simulink model "Simulink_Deliverable1_2__2_"  (R2025b)
settings: Solver=FixedStepAuto  StartTime=0.0  StopTime=10.0  FixedStep=1e-3  RelTol=1e-3  EnableMultiTasking=on
undefined symbols (not defined in the file): A0, A1, A2, A3, A4, D0, D1, D10, D11, D12, D13, D2, D3, D4, D5, D6, D7, D8, D9, PTA0, PTA1, PTA2, PTB10, PTB11, PTB2, PTB23, PTB3, PTB9, PTC11, PTC16, PTC17, PTC2, PTC3, PTC4, PTD0, PTD1, PTD2, PTD3
libraries: frdmk64flib x22, etargetslib x6, dspstat3 x2
settings Model: ExtModeTrigDuration=5  Creator=shaun  LastModifiedBy=anila
settings OptimizationCC: DefaultParameterBehavior=Inlined  EnhancedBackFolding=on  PassReuseOutputArgsAs=Individual arguments  ZeroExternalMemoryAtStartup=off  ZeroInternalMemoryAtStartup=off  MaxStackSize=64  OptimizeBlockOrder=speed  DifferentSizesBufferReuse=on  OptimizationCustomize=off  EfficientTunableParamExpr=on
settings DebuggingCC: ParameterTunabilityLossMsg=error
settings HardwareCC: ProdBitPerPointer=32.0  ProdBitPerSizeT=32.0  ProdBitPerPtrDiffT=32.0  ProdLargestAtomicInteger=Long  ProdLargestAtomicFloat=Double  ProdWordSize=32.0  ProdHWDeviceType=ARM Compatible->ARM Cortex
settings SFSimCC: MATLABDynamicMemAlloc=off
settings RTWCC: SystemTargetFile=ert.tlc  HardwareBoard=NXP FRDM-K64F  TLCOptions="-aInlineSetEventsForThisBaseRateFcn=TLC_FALSE -aSuppressMultiTaskScheduler=TLC_FALSE  -aRateBasedStepFcn=0"  TemplateMakefile=ert_default_tmf  Toolchain=GNU Tools for ARM Embedded Processors  Description=Embedded Coder
settings CodeAppCC: ForceParamTrailComments=on  IgnoreCustomStorageClasses=off  OperatorAnnotations=on  SimulinkDataObjDesc=on  SFDataObjDesc=on  InsertBlockDesc=on
settings ERTTargetCC: ExtModeTransport=4.0  ExtModeMexFile=sendToCommService

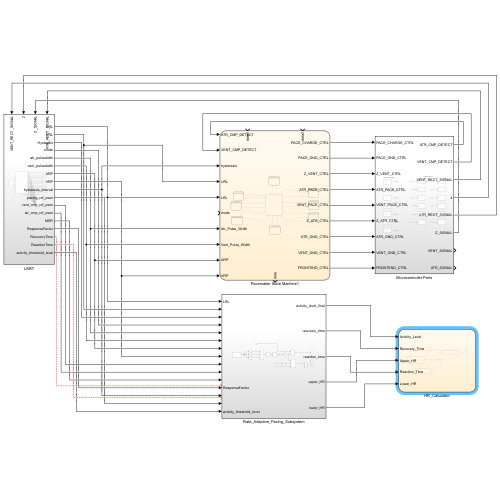
[thumbnail: Simulink's stored preview of the top-level diagram]
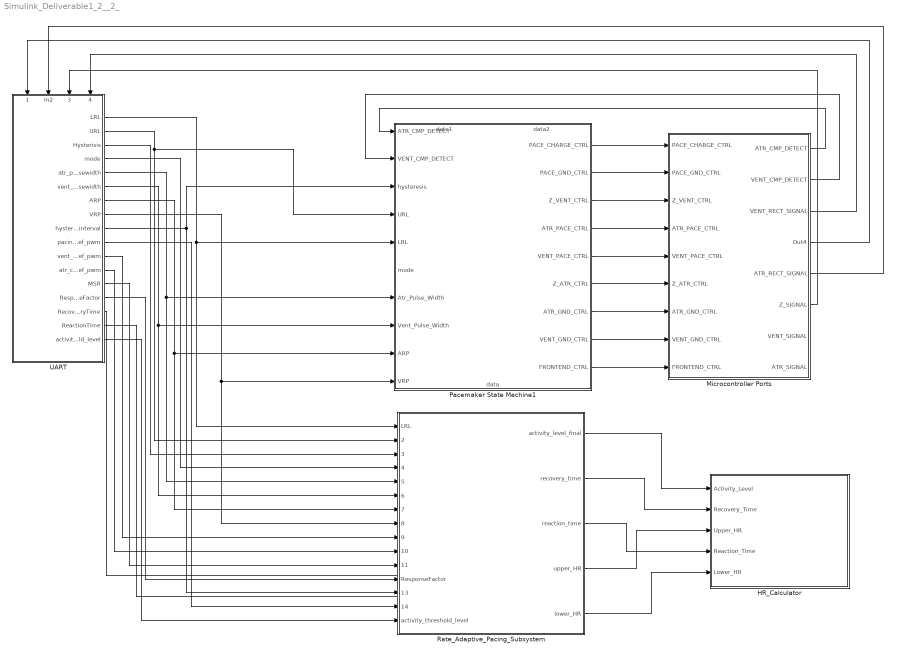
== system Simulink_Deliverable1_2__2_ ==
  HR_Calculator : Stateflow chart  TreatAsAtomicUnit=on
      settings: PortSchema="{\"entries\":[{\"content\":{\"sides\":[{\"content\":{\"connectorIds\":[\"In5\",\"In2\",\"In3\",\"In4\",\"In1\"]},\"type\":\"ConnectorPlacement.EquallySpacedRectSide\",\"uuid\":\"4fd71a97-0d96-44cf-9a3b-b475d577ae04\"},{\"content\":{\"side\":\"RIGHT\"},\"type\":\"ConnectorPlacement.EquallySpacedRectSide\",\"uuid\":\"faba256d-fac9-4ab5-bd75-12f2978d4ab7\"},{\"content\":{\"side\":\"TOP\"},\"type\":\"ConnectorPlacement.EquallySpacedRectSide\",\"uuid\":\"a02d704a-be11-4cb0-b416-0f22440acd8a\"}]},\"type\":\"ConnectorPlacement.EquallySpacedConnector\",\"uuid\":\"fcc24184-24f4-4090-bbbe-791745e2298d\"}],\"packageUris\":[\"http://schema.mathworks.com/mf0/Connector/R2020b\"],\"version\":\"1.0\"}"
  Microcontroller Ports : Subsystem
  Pacemaker State Machine1 : Stateflow chart  TreatAsAtomicUnit=on
      settings: PortSchema="{\"entries\":[{\"content\":{\"sides\":[{\"content\":{\"connectorIds\":[\"In4\",\"In11\",\"In3\",\"In5\",\"In6\",\"In9\",\"In7\",\"In10\",\"In8\",\"In12\"]},\"type\":\"ConnectorPlacement.EquallySpacedRectSide\",\"uuid\":\"3d18841d-ac72-4031-8466-622516bc8e89\"},{\"content\":{\"connectorIds\":[\"Out5\",\"Out6\",\"Out10\",\"Out3\",\"Out8\",\"Out9\",\"Out2\",\"Out7\",\"Out4\"],\"side\":\"RIGHT\"},\"type\":\"ConnectorPlacement.EquallySpacedRectSide\",\"uuid\":\"4d13c4f7-6767-44e3-9325-4ac8cd89e11a\"},{\"content\":{\"connectorIds\":[\"In1\",\"In2\"],\"side\":\"TOP\"},\"type\":\"ConnectorPlacement.EquallySpacedRectSide\",\"uuid\":\"87410120-6407-4e47-b91e-6c9b7b921b96\"},{\"content\":{\"connectorIds\":[\"Out1\"],\"side\":\"BOTTOM\"},\"type\":\"ConnectorPlacement.EquallySpacedRectSide\",\"uuid\":\"b376cdcd-045a-4cf2-9c04-75ec87224bb6\"}]},\"type\":\"ConnectorPlacement.EquallySpacedConnector\",\"uuid\":\"fed7b079-bf69-4c2d-9ed3-910cc0ad36be\"}],\"packageUris\":[\"http://schema.mathworks.com/mf0/Connector/R2020b\"],\"version\":\"1.0\"}"
  Rate_Adaptive_Pacing_Subsystem : Subsystem
  UART : Subsystem
      settings: PortSchema="{\"entries\":[{\"content\":{\"sides\":[{\"content\":{},\"type\":\"ConnectorPlacement.EquallySpacedRectSide\",\"uuid\":\"183065aa-c741-4563-b5ae-3020154dfd83\"},{\"content\":{\"connectorIds\":[\"Out1\",\"Out2\",\"Out3\",\"Out4\",\"Out5\",\"Out6\",\"Out7\",\"Out8\",\"Out9\",\"Out10\",\"Out11\",\"Out12\",\"Out13\",\"Out14\",\"Out15\",\"Out16\",\"Out17\"],\"side\":\"RIGHT\"},\"type\":\"ConnectorPlacement.EquallySpacedRectSide\",\"uuid\":\"65727c57-e161-4cba-a0e8-016175ec1656\"},{\"content\":{\"connectorIds\":[\"In1\",\"In2\",\"In3\",\"In4\"],\"side\":\"TOP\"},\"type\":\"ConnectorPlacement.EquallySpacedRectSide\",\"uuid\":\"c897ad8a-6ebd-4b90-9657-b8410c3521bd\"}]},\"type\":\"ConnectorPlacement.EquallySpacedConnector\",\"uuid\":\"08bd3836-6b13-4613-84df-35379265e920\"}],\"packageUris\":[\"http://schema.mathworks.com/mf0/Connector/R2020b\"],\"version\":\"1.0\"}"
  wires:
  Microcontroller Ports/2(VENT_CMP_DETECT) -> Pacemaker State Machine1/11(VENT_CMP_DETECT)
  Pacemaker State Machine1/9(Z_ATR_CTRL) -> Microcontroller Ports/6(Z_ATR_CTRL)
  Pacemaker State Machine1/4(FRONTEND_CTRL) -> Microcontroller Ports/9(FRONTEND_CTRL)
  Pacemaker State Machine1/5(PACE_CHARGE_CTRL) -> Microcontroller Ports/1(PACE_CHARGE_CTRL)
  Pacemaker State Machine1/3(ATR_PACE_CTRL) -> Microcontroller Ports/4(ATR_PACE_CTRL)
  Pacemaker State Machine1/2(ATR_GND_CTRL) -> Microcontroller Ports/7(ATR_GND_CTRL)
  Microcontroller Ports/1(ATR_CMP_DETECT) -> Pacemaker State Machine1/4(ATR_CMP_DETECT)
  Pacemaker State Machine1/8(VENT_PACE_CTRL) -> Microcontroller Ports/5(VENT_PACE_CTRL)
  Pacemaker State Machine1/6(PACE_GND_CTRL) -> Microcontroller Ports/2(PACE_GND_CTRL)
  Pacemaker State Machine1/10(Z_VENT_CTRL) -> Microcontroller Ports/3(Z_VENT_CTRL)
  Pacemaker State Machine1/7(VENT_GND_CTRL) -> Microcontroller Ports/8(VENT_GND_CTRL)
  UART/7(ARP) -> Pacemaker State Machine1/8(ARP), Rate_Adaptive_Pacing_Subsystem/7
  UART/5(atr_pulsewidth) -> Pacemaker State Machine1/7(Atr_Pulse_Width), Rate_Adaptive_Pacing_Subsystem/5
  UART/17(activity_threshold_level) -> Rate_Adaptive_Pacing_Subsystem/15(activity_threshold_level)
  UART/14(ResponseFactor) -> Rate_Adaptive_Pacing_Subsystem/12(ResponseFactor)
  UART/1(LRL) -> Pacemaker State Machine1/6(LRL), Rate_Adaptive_Pacing_Subsystem/1(LRL)
  UART/15(RecoveryTime) -> ?
  UART/16(ReactionTime) -> ?
  UART/2(URL) -> Pacemaker State Machine1/5(URL), Rate_Adaptive_Pacing_Subsystem/2
  UART/3(Hysterisis) -> Rate_Adaptive_Pacing_Subsystem/3
  UART/4(mode) -> Rate_Adaptive_Pacing_Subsystem/4
  UART/6(vent_pulsewidth) -> Pacemaker State Machine1/10(Vent_Pulse_Width), Rate_Adaptive_Pacing_Subsystem/6
  UART/8(VRP) -> Pacemaker State Machine1/12(VRP), Rate_Adaptive_Pacing_Subsystem/8
  UART/9(hysteresis_interval) -> Pacemaker State Machine1/3(hysteresis), Rate_Adaptive_Pacing_Subsystem/13
  UART/10(pacing_ref_pwm) -> Rate_Adaptive_Pacing_Subsystem/14
  UART/11(vent_cmp_ref_pwm) -> Rate_Adaptive_Pacing_Subsystem/9
  UART/12(atr_cmp_ref_pwm) -> Rate_Adaptive_Pacing_Subsystem/10
  UART/13(MSR) -> Rate_Adaptive_Pacing_Subsystem/11
  Rate_Adaptive_Pacing_Subsystem/5(lower_HR) -> HR_Calculator/1(Lower_HR)
  Rate_Adaptive_Pacing_Subsystem/1(activity_level_final) -> HR_Calculator/5(Activity_Level)
  Rate_Adaptive_Pacing_Subsystem/2(recovery_time) -> HR_Calculator/2(Recovery_Time)
  Rate_Adaptive_Pacing_Subsystem/4(upper_HR) -> HR_Calculator/3(Upper_HR)
  Rate_Adaptive_Pacing_Subsystem/3(reaction_time) -> HR_Calculator/4(Reaction_Time)
  Microcontroller Ports/3(VENT_RECT_SIGNAL) -> UART/4(ATR_RECT_SIGNAL)
  Microcontroller Ports/4(Out4) -> UART/1(VENT_RECT_SIGNAL)
  Microcontroller Ports/5(ATR_RECT_SIGNAL) -> UART/2(In2)
  Microcontroller Ports/6(Z_SIGNAL) -> UART/3(Z_SIGNAL)

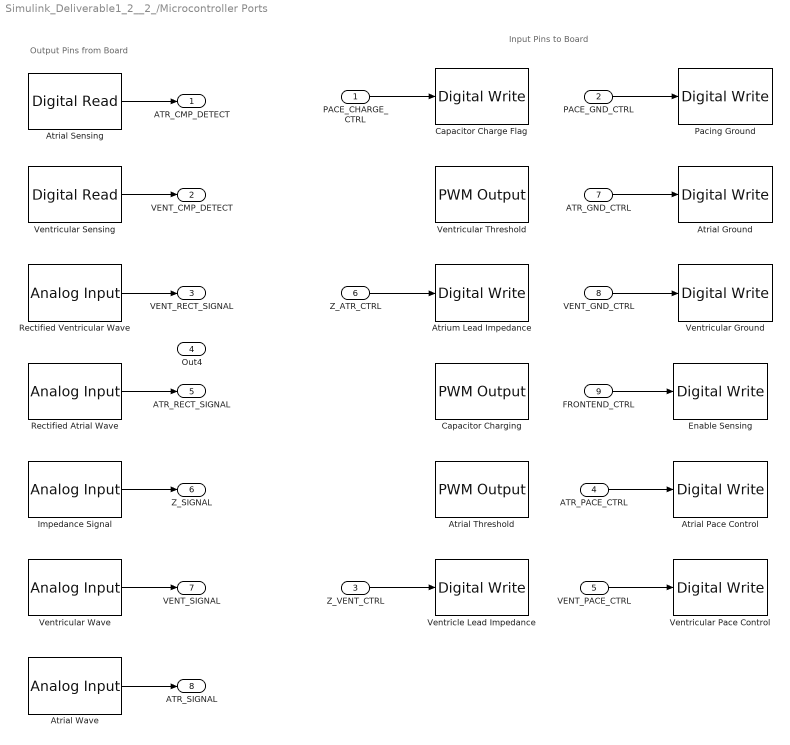
== system Simulink_Deliverable1_2__2_/Microcontroller Ports ==
  note: Output Pins from Board
  note: Input Pins to Board
  PACE_CHARGE_CTRL : Inport
  PACE_GND_CTRL : Inport  Port=2
  Z_VENT_CTRL : Inport  Port=3
  ATR_PACE_CTRL : Inport  Port=4
  VENT_PACE_CTRL : Inport  Port=5
  Z_ATR_CTRL : Inport  Port=6
  ATR_GND_CTRL : Inport  Port=7
  VENT_GND_CTRL : Inport  Port=8
  FRONTEND_CTRL : Inport  Port=9
  Atrial Ground : frdmk64flib/Digital Write  Whichpin=PTD2 (D11)
  Atrial Pace Control : frdmk64flib/Digital Write  Whichpin=PTA0 (D8)
  Atrial Sensing : frdmk64flib/Digital Read  Whichpin=PTC16 (D0)  SampleTime=-1
  Atrial Threshold : frdmk64flib/PWM Output  Whichpin=PTC2 (D6)  InitialFrequency=2000  InitialDutyCycle=0
  Atrial Wave : frdmk64flib/Analog Input  Whichpin=PTB2 (A0)  SampleTime=-1
  Atrium Lead Impedance : frdmk64flib/Digital Write  Whichpin=PTB23 (D4)
  Capacitor Charge Flag : frdmk64flib/Digital Write  Whichpin=PTB9 (D2)
  Capacitor Charging : frdmk64flib/PWM Output  Whichpin=PTA2 (D5)  InitialFrequency=2000  InitialDutyCycle=0
  Enable Sensing : frdmk64flib/Digital Write  Whichpin=PTD1 (D13)
  Impedance Signal : frdmk64flib/Analog Input  Whichpin=PTB10 (A2)  SampleTime=-1
  Pacing Ground : frdmk64flib/Digital Write  Whichpin=PTD0 (D10)
  Rectified Atrial Wave : frdmk64flib/Analog Input  Whichpin=PTB11 (A3)  SampleTime=-1
  Rectified Ventricular Wave : frdmk64flib/Analog Input  Whichpin=PTC11 (A4)  SampleTime=-1
  Ventricle Lead Impedance : frdmk64flib/Digital Write  Whichpin=PTC3 (D7)
  Ventricular Ground : frdmk64flib/Digital Write  Whichpin=PTD3 (D12)
  Ventricular Pace Control : frdmk64flib/Digital Write  Whichpin=PTC4 (D9)
  Ventricular Sensing : frdmk64flib/Digital Read  Whichpin=PTC17 (D1)  SampleTime=-1
  Ventricular Threshold : frdmk64flib/PWM Output  Whichpin=PTA1 (D3)  InitialFrequency=2000  InitialDutyCycle=0
  Ventricular Wave : frdmk64flib/Analog Input  Whichpin=PTB3 (A1)  SampleTime=-1
  ATR_CMP_DETECT : Outport
  VENT_CMP_DETECT : Outport  Port=2
  VENT_RECT_SIGNAL : Outport  Port=3
  Out4 : Outport  Port=4
  ATR_RECT_SIGNAL : Outport  Port=5
  Z_SIGNAL : Outport  Port=6
  VENT_SIGNAL : Outport  Port=7
  ATR_SIGNAL : Outport  Port=8
  wires:
  Atrial Sensing/1 -> ATR_CMP_DETECT/1
  Ventricular Sensing/1 -> VENT_CMP_DETECT/1
  PACE_CHARGE_CTRL/1 -> Capacitor Charge Flag/1
  ? -> Ventricular Threshold/1
  Z_ATR_CTRL/1 -> Atrium Lead Impedance/1
  ? -> Capacitor Charging/1
  ? -> Atrial Threshold/1
  Z_VENT_CTRL/1 -> Ventricle Lead Impedance/1
  ATR_PACE_CTRL/1 -> Atrial Pace Control/1
  VENT_PACE_CTRL/1 -> Ventricular Pace Control/1
  PACE_GND_CTRL/1 -> Pacing Ground/1
  ATR_GND_CTRL/1 -> Atrial Ground/1
  VENT_GND_CTRL/1 -> Ventricular Ground/1
  FRONTEND_CTRL/1 -> Enable Sensing/1
  Rectified Atrial Wave/1 -> ATR_RECT_SIGNAL/1
  Rectified Ventricular Wave/1 -> VENT_RECT_SIGNAL/1
  Impedance Signal/1 -> Z_SIGNAL/1
  Ventricular Wave/1 -> VENT_SIGNAL/1
  Atrial Wave/1 -> ATR_SIGNAL/1

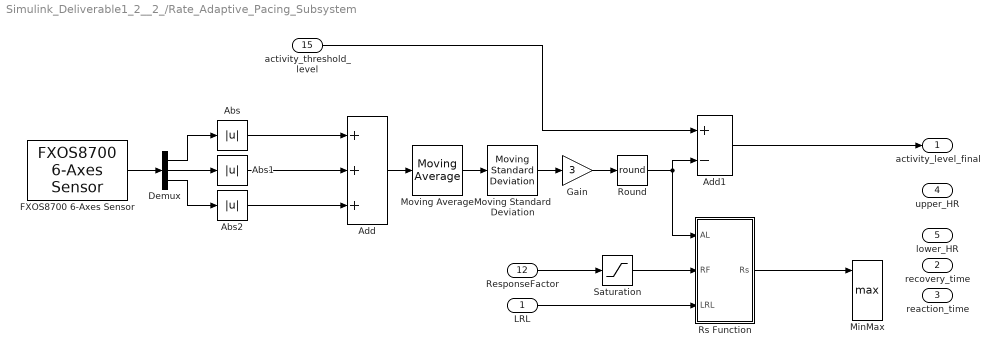
== system Simulink_Deliverable1_2__2_/Rate_Adaptive_Pacing_Subsystem ==
  LRL : Inport
  ResponseFactor : Inport  Port=12
  activity_threshold_level : Inport  Port=15
  Abs : Abs  SaturateOnIntegerOverflow=off
  Abs1 : Abs  SaturateOnIntegerOverflow=off
  Abs2 : Abs  SaturateOnIntegerOverflow=off
  Add : Sum  Inputs=+++
  Add1 : Sum  Inputs=+-
  Demux : Demux  Outputs=3
  FXOS8700 6-Axes Sensor : frdmk64flib/FXOS8700 6-Axes Sensor  Activesensor=Accelerometer only  ODR=800Hz  HybridODR=400Hz  Accelfullrange=-4g to +4g  SampleTime=-1
  Gain : Gain  Gain=3
  MinMax : MinMax  Function=max  Inputs=3
  Moving Average : dspstat3/Moving Average  Method=Sliding window  ForgettingFactorPort=off  SpecifyWindowLength=on  WindowLength=4  OverlapLength=3  AllowArbitraryInputLength=off  ForgettingFactor=0.9  SimulateUsing=Interpreted execution
  Moving Standard Deviation : dspstat3/Moving Standard Deviation  Method=Sliding window  ForgettingFactorPort=off  SpecifyWindowLength=on  WindowLength=4  OverlapLength=3  AllowArbitraryInputLength=off  ForgettingFactor=0.9  SimulateUsing=Interpreted execution
  Round : Rounding  Operator=round
  Rs Function : MATLAB Function  TreatAsAtomicUnit=on
  Saturation : Saturate  UpperLimit=14
  activity_level_final : Outport
  recovery_time : Outport  Port=2
  reaction_time : Outport  Port=3
  upper_HR : Outport  Port=4
  lower_HR : Outport  Port=5
  wires:
  FXOS8700 6-Axes Sensor/1 -> Demux/1
  Demux/1 -> Abs/1
  Demux/2 -> Abs1/1
  Demux/3 -> Abs2/1
  Abs/1 -> Add/1
  Abs1/1 -> Add/2
  Abs2/1 -> Add/3
  Add/1 -> Moving Average/1
  Moving Average/1 -> Moving Standard Deviation/1
  Moving Standard Deviation/1 -> Gain/1
  Gain/1 -> Round/1
  Round/1 -> Rs Function/1(AL), Add1/2
  LRL/1 -> Rs Function/3(LRL)
  Saturation/1 -> Rs Function/2(RF)
  ResponseFactor/1 -> Saturation/1
  activity_threshold_level/1 -> Add1/1
  Add1/1 -> activity_level_final/1
  Rs Function/1(Rs) -> MinMax/1

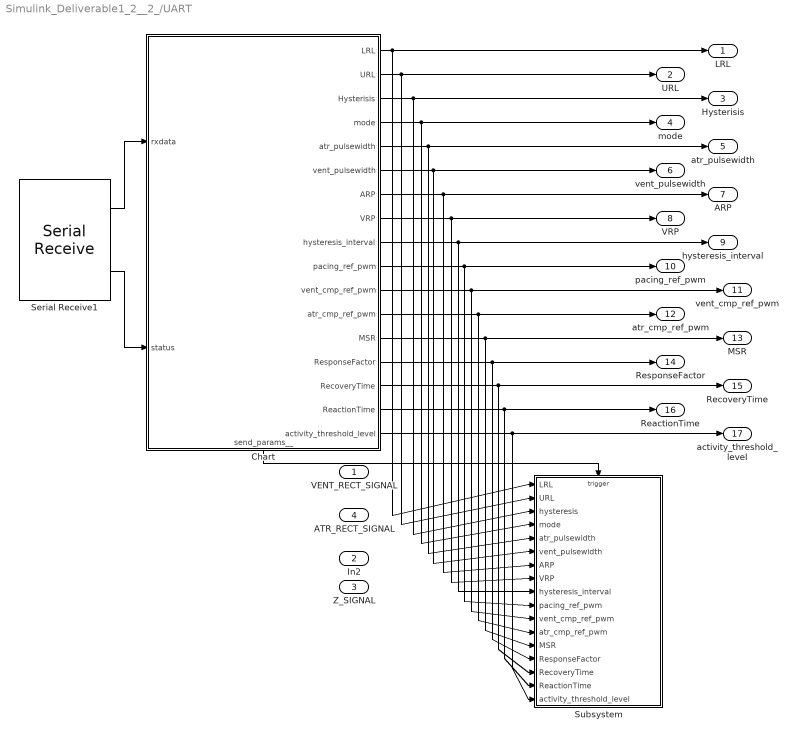
== system Simulink_Deliverable1_2__2_/UART ==
  VENT_RECT_SIGNAL : Inport
  In2 : Inport  Port=2
  Z_SIGNAL : Inport  Port=3
  ATR_RECT_SIGNAL : Inport  Port=4
  Chart : Stateflow chart  TreatAsAtomicUnit=on
      settings: PortSchema="{\"entries\":[{\"content\":{\"sides\":[{\"content\":{\"connectorIds\":[\"In1\",\"In2\"]},\"type\":\"ConnectorPlacement.EquallySpacedRectSide\",\"uuid\":\"bebe3e22-0960-44d0-8399-67e14216072d\"},{\"content\":{\"connectorIds\":[\"Out2\",\"Out3\",\"Out4\",\"Out5\",\"Out6\",\"Out7\",\"Out8\",\"Out9\",\"Out10\",\"Out11\",\"Out12\",\"Out13\",\"Out14\",\"Out15\",\"Out16\",\"Out17\",\"Out18\"],\"side\":\"RIGHT\"},\"type\":\"ConnectorPlacement.EquallySpacedRectSide\",\"uuid\":\"a4088612-4ea4-4c29-88bf-96f9d2b4fd9c\"},{\"content\":{\"side\":\"TOP\"},\"type\":\"ConnectorPlacement.EquallySpacedRectSide\",\"uuid\":\"7904bd59-2d39-416f-99c6-ab75130198a6\"},{\"content\":{\"connectorIds\":[\"Out1\"],\"side\":\"BOTTOM\"},\"type\":\"ConnectorPlacement.EquallySpacedRectSide\",\"uuid\":\"eb209d23-bc9c-4e28-840d-c030bd2810ba\"}]},\"type\":\"ConnectorPlacement.EquallySpacedConnector\",\"uuid\":\"1093a67f-4a83-45ff-8a38-c0bee63203db\"}],\"packageUris\":[\"http://schema.mathworks.com/mf0/Connector/R2020b\"],\"version\":\"1.0\"}"
  Serial Receive1 : frdmk64flib/Serial Receive  SCIModule=0  Baudrate=uint32(9600)  Parity=None  StopBits=1  HardwareFlowControl=None  ByteOrder=LittleEndian  DataType=uint8  DataLength=10  BlockingMode=off  OutputStatus=on  SampleTime=-1
  Subsystem : Subsystem
  LRL : Outport
  URL : Outport  Port=2
  Hysterisis : Outport  Port=3
  mode : Outport  Port=4
  atr_pulsewidth : Outport  Port=5
  vent_pulsewidth : Outport  Port=6
  ARP : Outport  Port=7
  VRP : Outport  Port=8
  hysteresis_interval : Outport  Port=9
  pacing_ref_pwm : Outport  Port=10
  vent_cmp_ref_pwm : Outport  Port=11
  atr_cmp_ref_pwm : Outport  Port=12
  MSR : Outport  Port=13
  ResponseFactor : Outport  Port=14
  RecoveryTime : Outport  Port=15
  ReactionTime : Outport  Port=16
  activity_threshold_level : Outport  Port=17
  wires:
  Serial Receive1/1 -> Chart/1(rxdata)
  Serial Receive1/2 -> Chart/2(status)
  Chart/2(LRL) -> LRL/1, Subsystem/1(LRL)
  Chart/3(URL) -> URL/1, Subsystem/2(URL)
  Chart/4(Hysterisis) -> Subsystem/3(hysteresis), Hysterisis/1
  Chart/5(mode) -> Subsystem/4(mode), mode/1
  Chart/6(atr_pulsewidth) -> Subsystem/5(atr_pulsewidth), atr_pulsewidth/1
  Chart/7(vent_pulsewidth) -> Subsystem/6(vent_pulsewidth), vent_pulsewidth/1
  Chart/8(ARP) -> Subsystem/7(ARP), ARP/1
  Chart/9(VRP) -> Subsystem/8(VRP), VRP/1
  Chart/10(hysteresis_interval) -> Subsystem/9(hysteresis_interval), hysteresis_interval/1
  Chart/11(pacing_ref_pwm) -> Subsystem/10(pacing_ref_pwm), pacing_ref_pwm/1
  Chart/12(vent_cmp_ref_pwm) -> Subsystem/11(vent_cmp_ref_pwm), vent_cmp_ref_pwm/1
  Chart/13(atr_cmp_ref_pwm) -> Subsystem/12(atr_cmp_ref_pwm), atr_cmp_ref_pwm/1
  Chart/14(MSR) -> Subsystem/13(MSR), MSR/1
  Chart/15(ResponseFactor) -> Subsystem/14(ResponseFactor), ResponseFactor/1
  Chart/16(RecoveryTime) -> Subsystem/15(RecoveryTime), RecoveryTime/1
  Chart/17(ReactionTime) -> Subsystem/16(ReactionTime), ReactionTime/1
  Chart/18(activity_threshold_level) -> Subsystem/17(activity_threshold_level), activity_threshold_level/1
  Chart/1(send_params__) -> Subsystem/Trigger

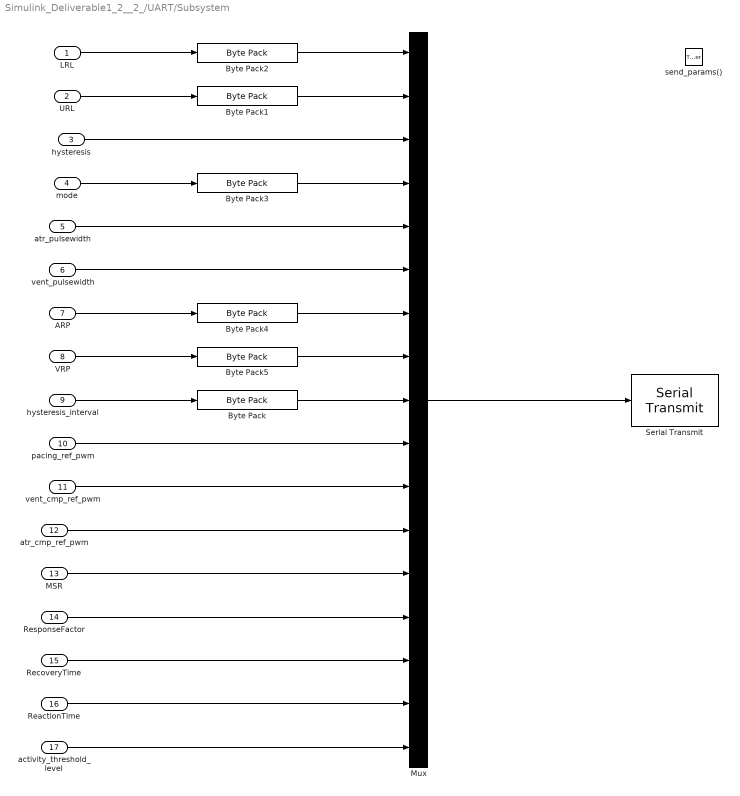
== system Simulink_Deliverable1_2__2_/UART/Subsystem ==
  LRL : Inport
  URL : Inport  Port=2
  hysteresis : Inport  Port=3
  mode : Inport  Port=4
  atr_pulsewidth : Inport  Port=5
  vent_pulsewidth : Inport  Port=6
  ARP : Inport  Port=7
  VRP : Inport  Port=8
  hysteresis_interval : Inport  Port=9
  pacing_ref_pwm : Inport  Port=10
  vent_cmp_ref_pwm : Inport  Port=11
  atr_cmp_ref_pwm : Inport  Port=12
  MSR : Inport  Port=13
  ResponseFactor : Inport  Port=14
  RecoveryTime : Inport  Port=15
  ReactionTime : Inport  Port=16
  activity_threshold_level : Inport  Port=17
  send_params() : TriggerPort  VariantControl=(inherit)  PortDimensions=1
  Byte Pack{,1..5} (6 alike) : etargetslib/Byte Pack  datatypes={'double'}  byteAlign=1
  Mux : Mux  Inputs=17
  Serial Transmit : frdmk64flib/Serial Transmit  SCIModule=0  Baudrate=uint32(9600)  Parity=None  StopBits=1  HardwareFlowControl=None  ByteOrder=LittleEndian  BlockingMode=on  OutputStatus=off
  wires:
  hysteresis/1 -> Mux/3
  atr_pulsewidth/1 -> Mux/5
  vent_pulsewidth/1 -> Mux/6
  pacing_ref_pwm/1 -> Mux/10
  vent_cmp_ref_pwm/1 -> Mux/11
  atr_cmp_ref_pwm/1 -> Mux/12
  MSR/1 -> Mux/13
  ResponseFactor/1 -> Mux/14
  RecoveryTime/1 -> Mux/15
  ReactionTime/1 -> Mux/16
  activity_threshold_level/1 -> Mux/17
  Mux/1 -> Serial Transmit/1
  Byte Pack/1 -> Mux/9
  hysteresis_interval/1 -> Byte Pack/1
  Byte Pack2/1 -> Mux/1
  LRL/1 -> Byte Pack2/1
  URL/1 -> Byte Pack1/1
  Byte Pack1/1 -> Mux/2
  mode/1 -> Byte Pack3/1
  Byte Pack3/1 -> Mux/4
  VRP/1 -> Byte Pack5/1
  Byte Pack5/1 -> Mux/8
  ARP/1 -> Byte Pack4/1
  Byte Pack4/1 -> Mux/7

== stateflow chart Simulink_Deliverable1_2__2_/Pacemaker State Machine1 ==
  state VOOR
    entry:
    state Initial_VOOR
      entry:
      %This is the initial state to define
      %varriables that wont change
      VOOR_amp = (p_vent_amplitude/5)*100;
      ATR_PACE_CTRL=0;
      ATR_GND_CTRL= 0;
      Z_ATR_CTRL=0;
      Z_VENT_CTRL=0;
    state Discharge_VOOR
      entry:
      %pacing state 3
      PACE_GND_CTRL=1;
      VENT_PACE_CTRL=0;
      VENT_GND_CTRL=1;
      %pacing state 1
      PACING_REF_PWM= VOOR_amp;
      PACE_CHARGE_CTRL=1;
    state Charge_VOOR
      entry:
      %pacing state 2
      PACE_CHARGE_CTRL=0;
      PACE_GND_CTRL=1;
      VENT_GND_CTRL=0;
      VENT_PACE_CTRL=1;
    (default) -> Initial_VOOR
    Initial_VOOR -> Discharge_VOOR
    Discharge_VOOR -> Charge_VOOR : [after(adaptive_time - p_vent_pw, msec)]
    Charge_VOOR -> Discharge_VOOR : [after(p_vent_pw, msec)]
  state AOO
    entry:
    state Discharge_AOO
      entry:
      %pacing state 3
      PACE_GND_CTRL=1;
      ATR_PACE_CTRL=0;
      ATR_GND_CTRL=1;
      %pacing state 1
      PACING_REF_PWM= AOO_amp;
      PACE_CHARGE_CTRL=1;
    state Initial_AOO
      entry:
      %Defining variables
      discharge_time = ((60/p_LRL)*1000)-p_atr_pw;
      AOO_amp = (p_atr_amplitude/5)*100;
      Z_VENT_CTRL=0;
      VENT_GND_CTRL=0;
      VENT_PACE_CTRL=0;
      Z_ATR_CTRL=0;
    state Charge_AOO
      entry:
      %pacing state 2
      PACE_CHARGE_CTRL=0;
      PACE_GND_CTRL=1;
      ATR_GND_CTRL= 0;
      ATR_PACE_CTRL=1;
    (default) -> Initial_AOO
    Initial_AOO -> Discharge_AOO
    Discharge_AOO -> Charge_AOO : [after(discharge_time, msec)]
    Charge_AOO -> Discharge_AOO : [after(p_atr_pw, msec)]
  state VOO
    entry:
    state Discharge_VOO
      entry:
      %pacing state 3
      PACE_GND_CTRL=1;
      VENT_PACE_CTRL=0;
      VENT_GND_CTRL=1;
      %pacing state 1
      PACING_REF_PWM= VOO_amp;
      PACE_CHARGE_CTRL=1;
    state Initial_VOO
      entry:
      %This is the initial state to define
      %varriables that wont change
      discharge_time = ((p_LRL/60)*1000)-p_vent_pw;
      VOO_amp = (p_vent_amplitude/5)*100;
      ATR_PACE_CTRL=0;
      ATR_GND_CTRL= 0;
      Z_ATR_CTRL=0;
      Z_VENT_CTRL=0;
    state Charge_VOO
      entry:
      %pacing state 2
      PACE_CHARGE_CTRL=0;
      PACE_GND_CTRL=1;
      VENT_GND_CTRL=0;
      VENT_PACE_CTRL=1;
    (default) -> Initial_VOO
    Initial_VOO -> Discharge_VOO
    Discharge_VOO -> Charge_VOO : [after(discharge_time, msec)]
    Charge_VOO -> Discharge_VOO : [after(p_vent_pw, msec)]
  state Initial_State
    entry:
    VENT_CMP_REF_PWM = 80;
    ATR_CMP_REF_PWM = 51;
  state AOOR
    entry:
    state Discharge_AOOR
      entry:
      %pacing state 3
      PACE_GND_CTRL=1;
      ATR_PACE_CTRL=0;
      ATR_GND_CTRL=1;
      %pacing state 1
      PACING_REF_PWM= AOOR_amp;
      PACE_CHARGE_CTRL=1;
    state Initial_AOOR
      entry:
      %Defining variables
      AOOR_amp = (p_atr_amplitude/5)*100;
      Z_VENT_CTRL=0;
      VENT_GND_CTRL=0;
      VENT_PACE_CTRL=0;
      Z_ATR_CTRL=0;
    state Charge_AOOR
      entry:
      %pacing state 2
      PACE_CHARGE_CTRL=0;
      PACE_GND_CTRL=1;
      ATR_GND_CTRL= 0;
      ATR_PACE_CTRL=1;
    (default) -> Initial_AOOR
    Initial_AOOR -> Discharge_AOOR
    Discharge_AOOR -> Charge_AOOR : [after(adaptive_time - p_atr_pw, msec)]
    Charge_AOOR -> Discharge_AOOR : [after(p_atr_pw, msec)]
  state VVIR
    entry:
    state Discharge_VVI
      entry:
      %pacing state 3
      PACE_GND_CTRL=1;
      VENT_PACE_CTRL=0;
      VENT_GND_CTRL=1;
      % pacing state 1
      PACING_REF_PWM= VVIR_amp;
      PACE_CHARGE_CTRL=1;
    state Initial_VVIR
      entry:
      %Initial state defining variables
      VVIR_amp = (p_vent_amplitude/5)*100;
      ATR_PACE_CTRL=0;
      ATR_GND_CTRL= 0;
      Z_ATR_CTRL=0;
      Z_VENT_CTRL=0;
    state Charge_VVIR
      entry:
      %pacing state 2
      PACE_CHARGE_CTRL=0;
      PACE_GND_CTRL=1;
      VENT_GND_CTRL=0;
      VENT_PACE_CTRL=1;
    (default) -> Initial_VVIR
    Initial_VVIR -> VVIR.Discharge_VVI
    VVIR.Discharge_VVI -> (junction 353)
    (junction 353) -> VVIR.Discharge_VVI [order 2] : [VENT_CMP_DETECT == true]
    Charge_VVIR -> VVIR.Discharge_VVI : [after(p_vent_pw, msec)]
    (junction 353) -> Charge_VVIR [order 1] : [after(adaptive_time - p_vent_pw, msec) && VENT_CMP_DETECT == false]
  state AAI
    entry:
    state Discharge_AAI
      entry:
      %pacing state 3
      PACE_GND_CTRL=1;
      ATR_PACE_CTRL=0;
      ATR_GND_CTRL=1;
      %pacing state 1
      PACING_REF_PWM= AAI_amp;
      PACE_CHARGE_CTRL=1;
    state Initial_AAI
      entry:
      %initial state defining variables
      discharge_time = ((60/p_LRL)*1000)-p_atr_pw;
      AAI_amp = (p_atr_amplitude/5)*100;
      Z_VENT_CTRL=0;
      VENT_GND_CTRL=0;
      VENT_PACE_CTRL=0;
      Z_ATR_CTRL=0;
    state Charge_AAI
      entry:
      %pacing state 2
      PACE_CHARGE_CTRL=0;
      PACE_GND_CTRL=1;
      ATR_GND_CTRL= 0;
      ATR_PACE_CTRL=1;
    (default) -> Initial_AAI
    Initial_AAI -> Discharge_AAI
    Discharge_AAI -> (junction 330)
    (junction 330) -> Discharge_AAI [order 2] : [ATR_CMP_DETECT == true]
    Charge_AAI -> Discharge_AAI : [after(p_atr_pw, msec)]
    (junction 330) -> Charge_AAI [order 1] : [after(discharge_time , msec) && ATR_CMP_DETECT == false]
  state VVI
    entry:
    state Discharge_VVI
      entry:
      %pacing state 3
      PACE_GND_CTRL=1;
      VENT_PACE_CTRL=0;
      VENT_GND_CTRL=1;
      % pacing state 1
      PACING_REF_PWM= VVI_amp;
      PACE_CHARGE_CTRL=1;
    state Initial_VVI
      entry:
      %Initial state defining variables
      discharge_time = ((60/p_LRL)*1000)-p_vent_pw;
      VVI_amp = (p_vent_amplitude/5)*100;
      ATR_PACE_CTRL=0;
      ATR_GND_CTRL= 0;
      Z_ATR_CTRL=0;
      Z_VENT_CTRL=0;
    state Charge_VVI
      entry:
      %pacing state 2
      PACE_CHARGE_CTRL=0;
      PACE_GND_CTRL=1;
      VENT_GND_CTRL=0;
      VENT_PACE_CTRL=1;
    (default) -> Initial_VVI
    Initial_VVI -> VVI.Discharge_VVI
    VVI.Discharge_VVI -> (junction 318)
    (junction 318) -> VVI.Discharge_VVI [order 2] : [VENT_CMP_DETECT == true]
    Charge_VVI -> VVI.Discharge_VVI : [after(p_vent_pw, msec)]
    (junction 318) -> Charge_VVI [order 1] : [after(discharge_time, msec) && VENT_CMP_DETECT == false]
  state AAIR
    entry:
    state Discharge_AAIR
      entry:
      %pacing state 3
      PACE_GND_CTRL=1;
      ATR_PACE_CTRL=0;
      ATR_GND_CTRL=1;
      %pacing state 1
      PACING_REF_PWM= AAIR_amp;
      PACE_CHARGE_CTRL=1;
    state Initial_AAIR
      entry:
      %initial state defining variables
      AAIR_amp = (p_atr_amplitude/5)*100;
      Z_VENT_CTRL=0;
      VENT_GND_CTRL=0;
      VENT_PACE_CTRL=0;
      Z_ATR_CTRL=0;
    state Charge_AAIR
      entry:
      %pacing state 2
      PACE_CHARGE_CTRL=0;
      PACE_GND_CTRL=1;
      ATR_GND_CTRL= 0;
      ATR_PACE_CTRL=1;
    (default) -> Initial_AAIR
    Initial_AAIR -> Discharge_AAIR
    Discharge_AAIR -> (junction 341)
    (junction 341) -> Discharge_AAIR [order 2] : [ATR_CMP_DETECT == true]
    Charge_AAIR -> Discharge_AAIR : [after(p_atr_pw, msec)]
    (junction 341) -> Charge_AAIR [order 1] : [after(adaptive_time -p_atr_pw , msec) && ATR_CMP_DETECT == false]
  Initial_State -> VOOR [order 2] : [p_pacing_mode == 5]
  VOOR -> Initial_State : [p_pacing_mode ~= 5]
  AOO -> Initial_State : [p_pacing_mode ~= 2]
  (default) -> Initial_State
  VOO -> Initial_State : [p_pacing_mode ~= 1]
  Initial_State -> AOO [order 6] : [p_pacing_mode == 2]
  Initial_State -> VOO [order 1] : [p_pacing_mode == 1]
  AOOR -> Initial_State : [p_pacing_mode ~= 6]
  Initial_State -> VVIR [order 3] : [p_pacing_mode == 8]
  Initial_State -> AOOR [order 5] : [p_pacing_mode == 6]
  VVIR -> Initial_State : [p_pacing_mode ~=  8]
  Initial_State -> VVI [order 8] : [p_pacing_mode == 4]
  Initial_State -> AAI [order 7] : [p_pacing_mode == 3]
  VVI -> Initial_State : [p_pacing_mode ~=  4]
  AAIR -> Initial_State : [p_pacing_mode ~= 7]
  Initial_State -> AAIR [order 4] : [p_pacing_mode == 7]
  AAI -> Initial_State : [p_pacing_mode ~= 3]
  data: data1 input; data2 input; data output; ATR_GND_CTRL output; ATR_PACE_CTRL output; FRONTEND_CTRL output; PACE_CHARGE_CTRL output; PACE_GND_CTRL output; VENT_GND_CTRL output; VENT_PACE_CTRL output; Z_ATR_CTRL output; Z_VENT_CTRL output; hysteresis input; ATR_CMP_DETECT input; URL input; LRL input; Atr_Pulse_Width input; ARP input; mode input; Vent_Pulse_Width input; VENT_CMP_DETECT input; VRP input

== matlab function Simulink_Deliverable1_2__2_/Rate_Adaptive_Pacing_Subsystem/Rs Function ==
  data: AL input; RF input; Rs output; LRL input
function Rs = fcn(AL, RF , LRL)

Rs = LRL + 4*RF*exp(AL+1);

== stateflow chart Simulink_Deliverable1_2__2_/UART/Chart ==
  state set_param__
    entry:
    LRL =
    URL
    hysteresis
  state Name
    entry:
    LRL = 60;
    URL = 120;
    hysteresis = 0;
    mode = 0;
    atr_pulsewidth = 0.4;
    vent_pulsewidth = 2;
    ARP = 250;
    VRP = 150;
    hysteresis_interval = 125;
    pacing_ref_pwm = 3.75;
    vent_cmp_ref_pwm = 3.5;
    atr_cmp_ref_pwm = 3.5;
    MSR = 120;
    ResponseFactor = 8;
    RecoveryTime = 5; %Minutes
    ReactionTime = 30; %Seconds
    activity_threshold_level = 3;
  state Standby
    %wait for coms
  state echo_params__
  (default) -> Name
  (junction 41) -> Standby : [2]
  Standby -> (junction 41) : [status == 0]
  echo_params__ -> (junction 46)
  Name -> Standby
  data: send_params__ output; rxdata input; status input; LRL output; URL output; Hysterisis output; mode output; atr_pulsewidth output; vent_pulsewidth output; ARP output; VRP output; hysteresis_interval output; pacing_ref_pwm output; vent_cmp_ref_pwm output; atr_cmp_ref_pwm output; MSR output; ResponseFactor output; RecoveryTime output; ReactionTime output; activity_threshold_level output

== stateflow chart Simulink_Deliverable1_2__2_/HR_Calculator ==
  state Reaction_Rate_Definition
    entry:
    reaction_Rate = (Upper_HR - curr_HR)/Reaction_Time;
    curr_Level = Activity_Level;
  state Increase_HR
    entry:
    curr_HR = curr_HR + reaction_Rate *d_time
  state Entry_State
    entry:
    curr_HR = Lower_HR;
    reaction_Rate = (Upper_HR - Lower_HR)/Reaction_Time;
    recovery_Rate = (Lower_HR - Upper_HR)/Recovery_Time;
    curr_Level = Activity_Level;
    d_time = 0.1;
  state Define_Recovery_Rate
    entry:
    curr_Level = Activity_Level;
    recovery_Rate = (Lower_HR - curr_HR)/Recovery_Time;
  Reaction_Rate_Definition -> (junction 19)
  (junction 25) -> (junction 19) [order 2] : [Activity_Level == curr_Level ]{after(d_time, sec)}
  (junction 25) -> (junction 48) [order 1] : [Activity_Level ~= curr_Level ]
  Increase_HR -> (junction 25)
  (junction 19) -> Increase_HR
  (junction 48) -> Reaction_Rate_Definition [order 2] : [Activity_Level > 0 ]{after(d_time,sec)}
  (default) -> Entry_State
  Entry_State -> (junction 48)
  (junction 48) -> Define_Recovery_Rate [order 1] : [Activity_Level <= 0]{after(d_time, sec)}
  Define_Recovery_Rate -> (junction 48)
  data: Lower_HR input; Recovery_Time input; Upper_HR input; Reaction_Time input; Activity_Level input; recovery_Rate local; reaction_Rate local; curr_Level local; d_time local
